simulink model "satellite_dynamics"  (R2025a)
settings: Solver=ode4  StartTime=0.0  StopTime=5400* 5  FixedStep=gyro.Ts  RelTol=1e-6
values from neighbouring files (symbols this model uses):
  altitude = 279e3    (= 279000)    [orbit_params.m]
  G = 6.674e-11    [orbit_params.m]    (also in update_MEKF_new.m = [-eye(3,3), zeros(3,3),zeros(3,3);          zeros(3,3), eye(; update_MEKF_old.m = [-eye(3,3), zeros(3,3);          zeros(3,3), eye(3,3)]; wheel_analysis.m = [ D)
  h_default = h_default + wheel.omega_initial(f) *  wheel.I_II * wheel.axes(:,f)    [orbit_params.m]
  K = convhulln(V)    [wheel_analysis.m]
  m = size(A, 2)    [wheel_analysis.m]
  omega_icrf2b_initial = [-0.3804;-0.2976;0.06] *0    [orbit_params.m]
  P_initial = blkdiag(eye(3) * gyro.sigma_v^2 * 1e4 ,eye(3) * gyro.sigma_u^2 * 1e5)    [orbit_params.m]
  Q_c = blkdiag(eye(3) * gyro.sigma_v^2/2 ,eye(3) * gyro.sigma_u^2/2 )    [orbit_params.m]
  q_icrf2b_initial = q_icrf2b_initial/norm(q_icrf2b_initial)    [orbit_params.m]
  q_initial = q_icrf2b_initial    [orbit_params.m]
  R_k_star = blkdiag(star.sigma_cross^2,star.sigma_cross^2,star.sigma_bore^2) * ((1/3600) * pi/180)^2    [orbit_params.m]
  r_offset = [1;1;5] * 1e-2    [orbit_params.m]
  regulation_kp = regulation.kp    [orbit_params.m]
  s = sign(h_bias)    [min_h.m]
  Ts = 0.1    [orbit_params.m]    (also in untitled2.m = 0.005)
  x_initial = zeros(6,1)    [orbit_params.m]
undefined symbols (not defined in the file or in its folder): DiscIntNeverNeededParam, earth, gyro, Kalman, mag, mag_torque, NEO, regulation, star, sun, tracking, wheel
libraries: utilities x24, simulink_extras x21, aerolibutil x20, dspmathops x19, matrix_library x9, simulink x8, dspstat3 x8, sharedutil x3, aerolibgravity2 x1, eeGeneralControl x1
(part 1 of 2)
settings Model: PacingRate=0.100000  Creator=OlguPilav  LastModifiedBy=OlguPilav

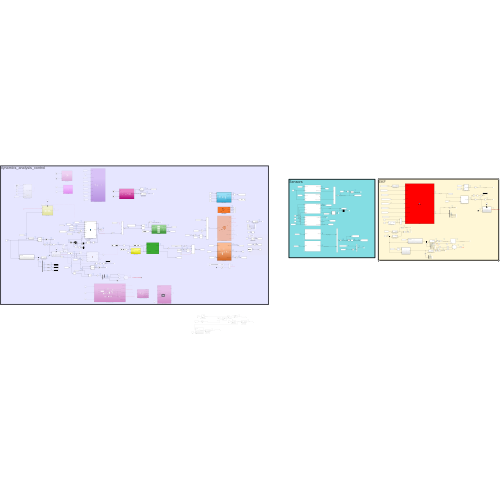
[thumbnail: Simulink's stored preview of the top-level diagram]
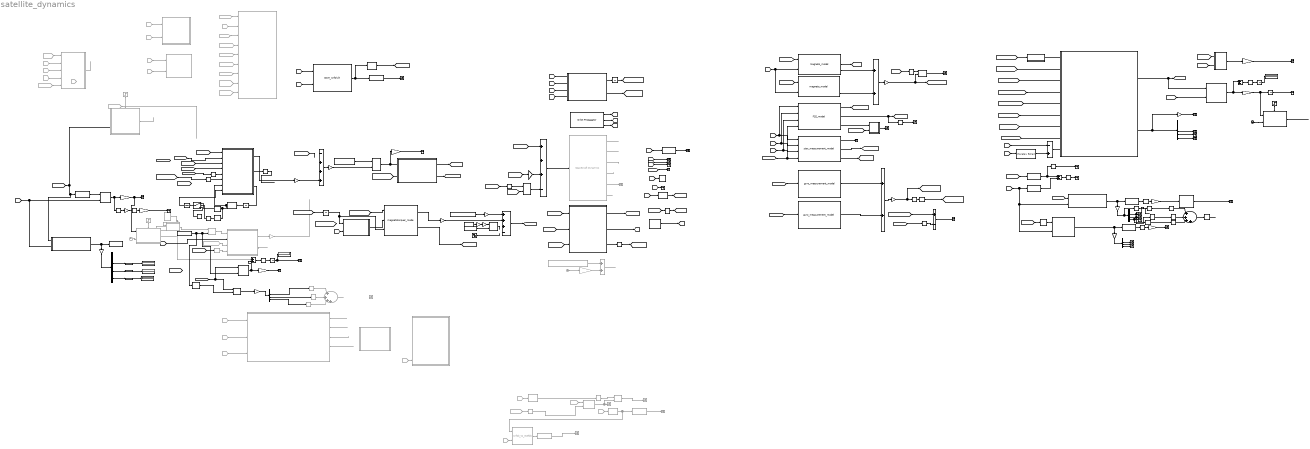
== system satellite_dynamics ==
  note: EKF
  note: Sensors
  note: dynamics_analysis_control
  Abs{,1..5} (6 alike) : Abs  SaturateOnIntegerOverflow=off
  Add : Sum
  Bias : Bias  Bias=gyro.bias  SaturateOnIntegerOverflow=off
  Clock : Clock  Commented=on
  Clock1 : Clock  Commented=on
  Clock2 : Clock
  Compare To Constant : simulink/Logic and Bit Operations/Compare To Constant  relop=>  const=0.999999  OutDataTypeStr=boolean
  Constant : Constant  Commented=on  Value=juliandate(year, month, day, hour, minute, second)
  Constant1 : Constant  Value=r_offset
  Constant2 : Constant  Value=q_icrf2b_initial
  Constant3 : Constant  Value=[0;0;0]
  Constant4 : Constant  Commented=on  Value=[1;1;1]
  Constant5 : Constant  Commented=on  Value=0
  Constant7 : Constant  Value=wheel.distribution_matrix
  Cross Product : matrix_library/Cross Product
  Cross Product1 : matrix_library/Cross Product
  DCM_icrf2lvlh : utilities/DCM_icrf2lvlh  SystemSampleTime=-1  VariantActivationTime=update diagram  EmptyChoice=off  PassThrough=off  PassThroughVariantControl=(default)  EmptyChoiceVariantControl=(default)  AllowFlexibleInterface=on  Latency=0  AutoFrameSizeCalculation=off
  Degrees to Radians : simulink_extras/Transformations/Degrees to Radians  Commented=on
  Degrees to Radians{1..6} (6 alike) : simulink_extras/Transformations/Degrees to Radians
  Degrees to Radians7 : simulink_extras/Transformations/Degrees to Radians  Commented=on
  Demux : Demux  Outputs=6
  Demux{1..4} (4 alike) : Demux
  Derivative : Derivative
  Direction Cosine Matrix to Rotation Angles : Dcm2Angle  Commented=on
      settings: AttributesFormatString=Rotation Order: %<rotationOrder>
  Direction Cosine Matrix to Rotation Angles1 : Dcm2Angle  Commented=on
      settings: AttributesFormatString=Rotation Order: %<rotationOrder>
  Direction Cosine Matrix to Rotation Angles2 : Dcm2Angle
      settings: AttributesFormatString=Rotation Order: %<rotationOrder>
  Direction Cosine Matrix to Quaternions : Dcm2Quat
  Direction Cosine Matrix to Quaternions1 : Dcm2Quat
  Discrete-Time Integrator : DiscreteIntegrator  SampleTime=-1  ICPrevOutput=DiscIntNeverNeededParam  ICPrevScaledInput=DiscIntNeverNeededParam
  Display{,1..4} (5 alike) : Display
  FSS_model : utilities/FSS_model  sun=sun
  Feedforward_torque_legacy : Subsystem  Commented=on
  From Workspace : FromWorkspace  VariableName=drag_simin
  From10 : From  Commented=on  GotoTag=omegaicrf2b_b
  From12 : From  Commented=on  GotoTag=tutc
  From13 : From  Commented=on  GotoTag=tutc
  From{14,20,43,83,96} (5 alike) : From  Commented=on  GotoTag=inertia
  From15 : From  Commented=on  GotoTag=Xicrf
  From{6,9,16,19,27..28,64} (7 alike) : From  Commented=on  GotoTag=qicrf2b
  From18 : From  Commented=on  GotoTag=omegaicrf2b_b
  From44 : From  Commented=on  GotoTag=Xicrf
  From45 : From  Commented=on  GotoTag=Vicrf
  From47 : From  Commented=on  GotoTag=DCMicrf2b
  From52 : From  Commented=on  GotoTag=DCMicrf2b
  From53 : From  Commented=on  GotoTag=hwheelsbody
  From{60..63} (4 alike) : From  Commented=on  GotoTag=dcmb2icrf
  From66 : From  Commented=on  GotoTag=Xicrf
  From84 : From  Commented=on  GotoTag=hwheelsbody
  From85 : From  Commented=on  GotoTag=q_icrf2b_kalman
  From93 : From  Commented=on  GotoTag=hwheelsbody
  Gain : Gain  Gain=0
  Gain1 : Gain  Gain=1/2
  Gain10 : Gain  Gain=3600 * 2 * 180/pi
  Gain11 : Gain  Gain=3600 * 2 * 180/pi
  Gain12 : Gain  Gain=1000
  Gain13 : Gain  Commented=on  Gain=1/86400
  Gain14 : Gain  Gain=3600 * 180/pi
  Gain15 : Gain  Gain=altitude
  Gain16 : Gain  Gain=1/2
  Gain17 : Gain  Gain=[-1;0;0]
  Gain18 : Gain  Gain=3600 * 2 * 180/pi
  Gain{2..3,6,8..9,19} (6 alike) : Gain  Gain=3600
  Gain20 : Gain  Gain=(2 * 180/pi) * 3600
  Gain21 : Gain  Commented=on
  Gain22 : Gain
  Gain23 : Gain  Gain=0
  Gain24 : Gain
  Gain4 : Gain  Gain=-1
  Gain5 : Gain  Gain=1/2
  Gain7 : Gain
  Integrator : Integrator
  Integrator1 : Integrator
  Integrator2 : Integrator
  MATLAB Function : MATLAB Function  Commented=on  TreatAsAtomicUnit=on
  MATLAB Function1 : MATLAB Function  TreatAsAtomicUnit=on
  MEKF : MATLAB Function  TreatAsAtomicUnit=on  SystemSampleTime=Kalman.Ts
  Matrix Multiply4 : Product  Multiplication=Matrix(*)
  Matrix Multiply7 : Product  Multiplication=Matrix(*)
  Matrix Multiply8 : Product  Commented=on  Multiplication=Matrix(*)
  Matrix Multiply9 : Product  Commented=on  Multiplication=Matrix(*)
  Moving Variance : dspstat3/Moving Variance  Method=Sliding window  ForgettingFactorPort=off  SpecifyWindowLength=on  WindowLength=20000  OverlapLength=19999  AllowArbitraryInputLength=off  ForgettingFactor=0.9  SimulateUsing=Interpreted execution
  Moving Variance1 : dspstat3/Moving Variance  Method=Sliding window  ForgettingFactorPort=off  SpecifyWindowLength=on  WindowLength=20000  OverlapLength=19999  AllowArbitraryInputLength=off  ForgettingFactor=0.9  SimulateUsing=Interpreted execution
  Moving Variance2 : dspstat3/Moving Variance  Method=Sliding window  ForgettingFactorPort=off  SpecifyWindowLength=on  WindowLength=20000  OverlapLength=19999  AllowArbitraryInputLength=off  ForgettingFactor=0.9  SimulateUsing=Interpreted execution
  Moving Averaage : Subsystem
  Orbit Propagator Kepler (unperturbed) : OrbitPropagator  startDate=juliandate(year, month, day, hour, minute, second)  semiMajorAxis=semi_major  eccentricity=eccentricity  inclination=inclination  raan=RAAN  argPeriapsis=periapsis_arg  trueAnomaly=true_anomaly  inertialPosition=[3649700.0 3308200.0 -4676600.0]  inertialVelocity=[-2750.8 6666.4 2573.4]  fixedPosition=[-4142689.0 -2676864.7 -4669861.6]  fixedVelocity=[1452.7 -6720.7 2568.1]  customR=3396200  customMu=4.305e13  customJ2=1.0826269e-03  customOmega=4.06125949e-3
  Planetary Ephemeris : PlanetaryEphem  units=m,m/s  target=Sun  outputVelocity=off
  Quaternion Inverse : aerolibutil/Quaternion Inverse
  Quaternion Inverse2 : aerolibutil/Quaternion Inverse
  Quaternion Multiplication : aerolibutil/Quaternion Multiplication  Commented=on
  Quaternion Multiplication1 : aerolibutil/Quaternion Multiplication
  Quaternions to Direction Cosine Matrix : Quat2Dcm  Commented=on
  Quaternions to Direction Cosine Matrix1 : Quat2Dcm
  Quaternions to Direction Cosine Matrix2 : Quat2Dcm  Commented=on
  Quaternions to Rotation Angles{,1..5} (6 alike) : Quat2Angle
      settings: AttributesFormatString=Rotation Order: %<rotationOrder>
  Radians to Degrees{,1..4} (5 alike) : simulink_extras/Transformations/Radians to Degrees
  Selector : Selector  InputPortWidth=4  IndexOptions=Index vector (dialog)  Indices=[2:4]  OutputSizes=1
  Selector1 : Selector  InputPortWidth=4  IndexOptions=Index vector (dialog)  Indices=[1]  OutputSizes=1
  Sine Wave : Sin  Amplitude=0.001  Frequency=6  SampleTime=0
  Spacecraft Dynamics : SpacecraftDynamics  Commented=on  forcesIn=off  startDate=juliandate(year, month, day, hour, minute, second)  mass=NEO.mass  inertia=NEO.inertia  semiMajorAxis=semi_major  eccentricity=eccentricity  inclination=inclination  raan=RAAN  argPeriapsis=periapsis_arg  trueAnomaly=true_anomaly  attitude=q_icrf2b_initial  attitudeRate=omega_icrf2b_initial  outputAngAccel=on  useGravGrad=off  useEOPs=off  useThirdBodyGravity=on  useSRP=on
  Sqrt : Sqrt
  Square : Math  Operator=square
  Square1 : Math  Operator=square
  Square2 : Math  Operator=square
  Square3 : Math  Commented=on  Operator=square
  Square4 : Math  Commented=on  Operator=square
  Square5 : Math  Commented=on  Operator=square
  Step : Step  Commented=on  SampleTime=0
  Step1 : Step  Commented=on  Time=1000  SampleTime=0
  Step2 : Step  Time=1000  SampleTime=0
  Subsystem : Subsystem  Commented=on
  Subsystem1 : Subsystem
  Subsystem2 : Subsystem  TreatAsAtomicUnit=on  SystemSampleTime=star.Ts
  Subsystem3 : Subsystem  TreatAsAtomicUnit=on  SystemSampleTime=Kalman.Ts
  Subsystem4 : Subsystem
  Subsystem6 : Subsystem  TreatAsAtomicUnit=on  SystemSampleTime=Kalman.Ts
  Subtract{,1,3..4} (4 alike) : Sum  Inputs=+-
  Subtract2 : Sum  Inputs=-+
  Sum : Sum
  Sum of Elements : Sum  Inputs=+
  Sum1 : Sum  Inputs=-+++
  Sum2 : Sum  Commented=on
  Sum3 : Sum  Inputs=|++++
  Sum4 : Sum  Commented=on  Inputs=|++++
  Sum6 : Sum  Inputs=+++-
  Sum7 : Sum  Inputs=+++-
  Switch : Switch  Criteria=u2 > Threshold  SaturateOnIntegerOverflow=off  InputSameDT=off
  Tan : Trigonometry  Operator=tan
  Terminator{,1..3,5..6,9..13,16..36,38} (33 alike) : Terminator
  Terminator{4,7..8,14..15,37} (6 alike) : Terminator  Commented=on
  Transpose2 : Math  Operator=transpose
  Transpose4 : Math  Operator=transpose
  Transpose5 : Math  Commented=on  Operator=transpose
  Unit Delay : UnitDelay  SampleTime=-1  HasFrameUpgradeWarning=on
  Unit Delay1 : UnitDelay  InitialCondition=[50,50,50]  SampleTime=-1  HasFrameUpgradeWarning=on
  Unit Delay2 : UnitDelay  InitialCondition=[50,50,50]  SampleTime=-1  HasFrameUpgradeWarning=on
  angular_momentum_calculations : Subsystem  Commented=on
  average_angle_knowledge_error : Subsystem  AncestorBlock=utilities/average_angle_knowledge_error  TreatAsAtomicUnit=on  SystemSampleTime=Kalman.Ts  mask{samples=2}
  average_angle_knowledge_error1 : Subsystem  AncestorBlock=utilities/average_angle_knowledge_error  TreatAsAtomicUnit=on  SystemSampleTime=star.Ts  mask{samples=2}
  average_angle_knowledge_error2 : utilities/average_angle_knowledge_error  samples=2
  average_angle_knowledge_error3 : utilities/average_angle_knowledge_error  samples=2
  disturbance : Constant  Value=[0.00001,0.00005,0.000]'  VectorParams1D=off
  earth_tracking_controller : MATLAB Function  TreatAsAtomicUnit=on
  geo_constrained_prograde aligned : Subsystem  Commented=on
  gyro_measurement_model : utilities/gyro_measurement_model  omega_initial=omega_icrf2b_initial  gyro=gyro
  gyro_measurement_model1 : utilities/gyro_measurement_model  omega_initial=omega_icrf2b_initial  gyro=gyro2
  icrf2b_to_ecef2b : utilities/icrf2b_to_ecef2b  Commented=on  SystemSampleTime=-1  VariantActivationTime=update diagram  EmptyChoice=off  PassThrough=off  PassThroughVariantControl=(default)  EmptyChoiceVariantControl=(default)  AllowFlexibleInterface=on  Latency=0  AutoFrameSizeCalculation=off
  inertia_b : Constant  Value=NEO.inertia
  magnetic_field_slow : Subsystem  TreatAsAtomicUnit=on  SystemSampleTime=60
  magneto_model : utilities/magneto_model  mag=mag
  magneto_model1 : utilities/magneto_model  mag=mag2
  magnetotorquer_mode : utilities/magnetotorquer_mode  Parameter1=mag_torque
  magtor_controller : Subsystem
  nadir_constrained_sun_aligned : Subsystem  Commented=on
  olgus_dynamics : Subsystem  TreatAsAtomicUnit=on  SystemSampleTime=Ts
  quat_tester : Subsystem  Commented=on
  quat_tester_2 : Subsystem  Commented=on
  regulating_controller : MATLAB Function  Commented=on  TreatAsAtomicUnit=on  SystemSampleTime=Kalman.Ts
  star_measurement_model : utilities/star_measurement_model  star=star
  target_q_generator : Subsystem  Commented=on
  vector_magnitude : utilities/vector_magnitude
  vector_magnitude1 : utilities/vector_magnitude
  wheel_controller : Subsystem  Commented=on  TreatAsAtomicUnit=on  SystemSampleTime=Kalman.Ts
  wheels_dynamics : Subsystem
  wires:
  Spacecraft Dynamics/5 -> Terminator4/1  "omega_dot_icrf2b"
  Quaternions to Direction Cosine Matrix/1 -> Direction Cosine Matrix to Rotation Angles/1, icrf2b_to_ecef2b/1  "DCM_icrf2b"
  icrf2b_to_ecef2b/1 -> Direction Cosine Matrix to Rotation Angles1/1
  Direction Cosine Matrix to Rotation Angles/1 -> Terminator7/1  "R_icrf2b"
  Direction Cosine Matrix to Rotation Angles1/1 -> Terminator8/1  "R_ecef2b"
  Spacecraft Dynamics/1 -> ?  "X_icrf"
  [Xicrf] -> Terminator/1
  Spacecraft Dynamics/2 -> ?  "V_icrf"
  [Vicrf] -> Terminator1/1
  Spacecraft Dynamics/3 -> ?  "q_icrf2b"
  [qicrf2b] -> Terminator2/1
  From6/1 -> Quaternions to Direction Cosine Matrix/1
  Spacecraft Dynamics/4 -> ?  "omega_icrf2b_b"
  [omegaicrf2b_b] -> Terminator3/1
  Spacecraft Dynamics/6 -> ?  "t_utc"
  [tutc] -> Terminator5/1
  From13/1 -> icrf2b_to_ecef2b/2
  inertia_b/1 -> [inertia]  "inertia"
  [qicrf2b] -> Quaternions to Direction Cosine Matrix1/1
  From19/1 -> Quaternions to Direction Cosine Matrix2/1
  Quaternions to Direction Cosine Matrix2/1 -> Transpose5/1  "DCM_icrf2b"
  From18/1 -> Degrees to Radians/1
  Matrix Multiply9/1 -> Matrix Multiply8/2, Terminator14/1  "h_body"
  Transpose5/1 -> Matrix Multiply8/1
  Matrix Multiply8/1 -> Terminator15/1  "h_icrf2"
  Degrees to Radians/1 -> Matrix Multiply9/2  "omega_body"
  From20/1 -> Matrix Multiply9/1
  [Xicrf] -> DCM_icrf2lvlh/1
  [Vicrf] -> DCM_icrf2lvlh/2
  DCM_icrf2lvlh/1 -> Direction Cosine Matrix to Quaternions/1, Direction Cosine Matrix to Rotation Angles2/1  "DCM_icrf2lvlh"
  Direction Cosine Matrix to Rotation Angles2/1 -> Terminator6/1  "R_LVLH"
  [qicrf2b] -> Quaternions to Rotation Angles/1
  Quaternions to Rotation Angles/1 -> Terminator9/1  "R_icrf"
  Direction Cosine Matrix to Quaternions/1 -> [qicrf2lvlh]  "q_icrf2lvlh"
  From16/1 -> nadir_constrained_sun_aligned/2(In2)
  From15/1 -> nadir_constrained_sun_aligned/1(In1)
  From12/1 -> nadir_constrained_sun_aligned/3(In3)
  nadir_constrained_sun_aligned/1(tar_primary_icrf) -> ?
  nadir_constrained_sun_aligned/2(tar_secondary_icrf) -> ?
  nadir_constrained_sun_aligned/3(body_primary_icrf) -> ?
  nadir_constrained_sun_aligned/4(body_secondary_icrf) -> ?
  From9/1 -> target_q_generator/5(qicrf2b)
  [qicrf2b] -> vector_magnitude1/1
  olgus_dynamics/1(omega_icrf2b_b) -> [omegaicrf2b_b]  "omega_icrf2b_b_new"
  olgus_dynamics/2(q_icrf2b) -> [qicrf2b]  "q_icrf2b"
  [omegaicrf2b_b] -> gyro_measurement_model/1
  gyro_measurement_model/1 -> Sum/1  "omega_icrf2b_gyro"
  [Xicrf] -> star_measurement_model/2, FSS_model/2
  [tutc] -> FSS_model/3, star_measurement_model/3
  star_measurement_model/1 -> Terminator13/1  "q_icrf2star_meas"
  [qicrf2b] -> FSS_model/1, star_measurement_model/1
  [omegaicrf2b_b] -> gyro_measurement_model1/1
  gyro_measurement_model1/1 -> Sum/2  "omega_icrf2b_gyro2"
  Sum/1 -> Gain1/1
  Gain1/1 -> [omega_gyro_pre_bias_degree], Degrees to Radians3/1  "omega_icrf2b_gyro_mean"
  MEKF/1(q_k_k) -> average_angle_knowledge_error/1(q_1), [q_icrf2b_kalman]  "q_icrf2b_kalman"
  MEKF/2(x_k_k) -> Gain14/1, Demux/1  "x_kalman"
  [omegaicrf2b_b] -> Degrees to Radians4/1
  Degrees to Radians4/1 -> Subtract1/2
  Subtract1/1 -> ?  "bias"
  Demux/4 -> Terminator26/1  "bias_kalman_1"
  Demux/5 -> Terminator28/1  "bias_kalman_2"
  Demux/6 -> Terminator27/1  "bias_kalman_3"
  [qicrf2b] -> average_angle_knowledge_error/2(q_2)
  average_angle_knowledge_error/1(error_degrees) -> Subtract4/1, Gain3/1  "error_kalman"
  [qicrf2b] -> average_angle_knowledge_error1/2(q_2)
  average_angle_knowledge_error1/1(error_degrees) -> Gain2/1  "error_star"
  Gain3/1 -> Subsystem4/1(In1), Integrator1/1  "error_kalman_arcsec"
  Gain2/1 -> Terminator18/1  "error_star_arcsec"
  Integrator1/1 -> Terminator16/1  "integral_kalman_error"
  [Xicrf] -> Subtract2/1
  [tutc] -> Planetary Ephemeris/1
  Planetary Ephemeris/1 -> Subtract2/2  "sun_icrf"
  Subtract2/1 -> MEKF/9(sat2sun_icrf)  "sat2sun_icrf"
  Sum of Elements/1 -> Terminator24/1
  [qicrf2b] -> magneto_model1/2, magneto_model/2
  magneto_model/3 -> Add/1
  magneto_model1/3 -> Add/2
  Add/1 -> Gain5/1
  Gain5/1 -> Matrix Multiply4/2, [magXYZbodymeasavg]  "mag_XYZ_body_meas_avg"
  [DCMicrf2b] -> Transpose2/1
  Transpose2/1 -> Matrix Multiply4/1
  Matrix Multiply4/1 -> Terminator11/1  "mag_XYZ_icrf_meas_avg"
  Gain6/1 -> Subsystem/1(In1), Terminator21/1  "error_target_arcsec"
  average_angle_knowledge_error2/1 -> Degrees to Radians1/1, Gain6/1  "error_target"
  earth_tracking_controller/1(torque) -> Gain24/1
  Sum1/1 -> Gain7/1
  Quaternions to Rotation Angles1/1 -> Subtract3/1, Radians to Degrees1/1
  Quaternions to Rotation Angles2/1 -> Subtract3/2
  Subtract3/1 -> Radians to Degrees/1
  Radians to Degrees/1 -> Terminator17/1
  Radians to Degrees1/1 -> Terminator19/1  "rot_angles_est"
  Gain7/1 -> Matrix Multiply7/2
  Degrees to Radians3/1 -> Bias/1
  Quaternions to Rotation Angles3/1 -> Radians to Degrees2/1  "rot_errors"
  Gain8/1 -> vector_magnitude/1  "rot_errors_kalman_arcsec"
  Radians to Degrees2/1 -> Gain8/1
  Quaternions to Rotation Angles4/1 -> Radians to Degrees3/1
  Gain9/1 -> Terminator31/1  "rot_errors_star_arcsec"
  [qicrf2b] -> Quaternions to Rotation Angles2/1, Subsystem2/2(r), Subsystem3/2(r)
  Radians to Degrees3/1 -> Gain9/1
  Demux2/4 -> Terminator35/1  "z_star"
  Demux3/2 -> Abs1/1, Terminator29/1  "x_k"
  Demux3/3 -> Abs2/1, Terminator30/1  "y_k"
  Demux3/4 -> Abs3/1, Terminator32/1  "z_k"
  Demux2/3 -> Terminator34/1  "y_star"
  Demux2/2 -> Terminator33/1  "x_star"
  Gain10/1 -> Abs/1, Demux3/1
  Gain11/1 -> Demux2/1
  Subsystem2/1(q*r) -> Gain11/1, Quaternions to Rotation Angles4/1
  Quaternion Inverse2/1 -> Subsystem2/1(q)
  Subsystem3/1(q*r) -> Quaternions to Rotation Angles3/1, Gain10/1
  Moving Averaage/1(omega_movav) -> MEKF/1(omega_icrf2b_gyro)
  FSS_model/2 -> [FSSvalid], Sum of Elements/1  "FSS_valid"
  Gain14/1 -> Terminator12/1  "x_kalman_arcsec"
  vector_magnitude/1 -> Terminator25/1  "mag_error_kalman_rot"
  FSS_model/3 -> MATLAB Function1/1(b1)
  MATLAB Function1/1(y) -> Terminator23/1  "vars"
  Constant7/1 -> Matrix Multiply7/1
  Matrix Multiply7/1 -> Gain12/1, wheels_dynamics/1(wheel_torques)
  [omega_dot_body] -> wheels_dynamics/2(satellite_body_omega_dot)
  Gain4/1 -> Sum6/3
  Gain12/1 -> Terminator20/1  "wheel_torques_demand_mNm"
  olgus_dynamics/3(omega_dot_icrf2b_b) -> Degrees to Radians5/1
  Degrees to Radians5/1 -> [omega_dot_body]
  Step/1 -> wheel_controller/Enable
  ? -> wheel_controller/1(qicrf2b)
  Subsystem1/1(q_out) -> average_angle_knowledge_error2/1
  Sum6/1 -> Spacecraft Dynamics/1
  Cross Product1/1 -> Sum6/4
  Degrees to Radians2/1 -> Cross Product1/1
  [mag_XYZ_b_model] -> magnetotorquer_mode/1
  magnetotorquer_mode/1 -> Gain23/1
  magtor_controller/1(currents) -> magnetotorquer_mode/2
  [magXYZbodymeasavg] -> Unit Delay2/1
  disturbance/1 -> Gain/1
  Gain/1 -> Sum7/1
  wheels_dynamics/2(angular_momentum_body) -> [hwheelsbody]  "h_wheels_body"
  [hwheelsbody] -> Cross Product1/2
  [hwheelsbody] -> olgus_dynamics/2(h_wheels_body)
  [hwheelsbody] -> magtor_controller/2(h_wheels_body)
  From44/1 -> Feedforward_torque_legacy/2(Xicrf)
  From45/1 -> Feedforward_torque_legacy/3(Vicrf)
  Feedforward_torque_legacy/1(target_torque) -> ?
  Quaternions to Direction Cosine Matrix1/1 -> [DCMicrf2b]  "DCM_icrf2b"
  [DCMicrf2b] -> Transpose4/1
  From52/1 -> Feedforward_torque_legacy/1(DCM_icrf2b)
  wheels_dynamics/1(body_torque) -> [wheelsbodytorque]  "wheels_body_torque"
  [wheelsbodytorque] -> olgus_dynamics/1(Mb_wheel)
  [wheelsbodytorque] -> Gain4/1
  Sum7/1 -> [Mbexternal]  "Mb_external"
  [Mbexternal] -> olgus_dynamics/3(Mb_external)
  [Mbexternal] -> Sum6/1
  [omegaicrf2b_b] -> Degrees to Radians2/1
  Transpose4/1 -> [dcmb2icrf]  "dcm_b2icrf"
  From28/1 -> quat_tester/1(q)
  From64/1 -> quat_tester/2(In2)
  From62/1 -> angular_momentum_calculations/1(dcmb2icrf)
  From43/1 -> angular_momentum_calculations/2(inertia)
  From10/1 -> angular_momentum_calculations/3(omegaicrf2b_b)
  From60/1 -> angular_momentum_calculations/4(dcmb2icrf2)
  From14/1 -> angular_momentum_calculations/5(inertia2)
  From47/1 -> angular_momentum_calculations/6(DCMicrf2b)
  From63/1 -> angular_momentum_calculations/7(dcmb2icrf3)
  From61/1 -> angular_momentum_calculations/8(dcmb2icrf4)
  From53/1 -> angular_momentum_calculations/9(hwheelsbody)
  From27/1 -> quat_tester_2/1(In1)
  From66/1 -> quat_tester_2/2(X_icrf)
  [magXYZicrfmodel] -> MATLAB Function1/2(b2)
  [magXYZicrfmodel] -> MEKF/6(mag_XYZ_icrf_model)
  [magXYZicrfmodel] -> magneto_model1/1
  [magXYZicrfmodel] -> magneto_model/1
  Bias/1 -> [omegaicrf2bgyromeanrad]  "omega_icrf2b_gyro_mean_rad"
  [omegaicrf2bgyromeanrad] -> Moving Averaage/1(omega_in)
  [omegaicrf2bgyromeanrad] -> Subtract1/1
  magneto_model/2 -> [magvalid]  "mag_valid"
  [magvalid] -> MEKF/8(mag_valid)
  [magXYZbodymeasavg] -> MEKF/7(mag_XYZ_body_meas)
  FSS_model/1 -> [sat2sunbody]  "sat2sun_body"
  [sat2sunbody] -> MEKF/4(sun_vectors)
  [FSSvalid] -> MEKF/5(sun_valid)
  star_measurement_model/3 -> [qicrf2bstartracker]  "q_icrf2b_star_tracker"
  [qicrf2bstartracker] -> MEKF/2(q_icrf2b_star)
  [qicrf2bstartracker] -> average_angle_knowledge_error1/1(q_1)
  [qicrf2bstartracker] -> Quaternion Inverse2/1
  [q_icrf2b_kalman] -> Quaternions to Rotation Angles1/1
  [q_icrf2b_kalman] -> Subsystem3/1(q_icrf2b_kalman)
  From83/1 -> Feedforward_torque_legacy/4(inertia)
  From84/1 -> Feedforward_torque_legacy/5(hwheelsbody)
  [qicrf2b] -> magnetic_field_slow/1(In1)
  [Xicrf] -> magnetic_field_slow/2(vector_icrf)
  [tutc] -> magnetic_field_slow/3(t_utc)
  [tutc] -> magnetic_field_slow/4(t_utc1)
  magnetic_field_slow/1(mag_XYZ_b_model) -> Unit Delay1/1
  magnetic_field_slow/2(mag_XYZ_icrf_model) -> [magXYZicrfmodel]
  Clock/1 -> Gain13/1
  Sum2/1 -> ?
  Gain13/1 -> Sum2/2
  Constant/1 -> Sum2/1
  Orbit Propagator Kepler (unperturbed)/1 -> [Xicrf]  "X_icrf"
  Orbit Propagator Kepler (unperturbed)/2 -> [Vicrf]  "V_icrf"
  Orbit Propagator Kepler (unperturbed)/3 -> [tutc]
  Degrees to Radians1/1 -> Gain16/1
  Tan/1 -> Gain15/1
  Gain15/1 -> Terminator36/1  "error_geo_meter"
  Gain16/1 -> Tan/1
  star_measurement_model/2 -> [STARVALID]  "STAR_VALID"
  [STARVALID] -> MEKF/3(star_valid)
  Cross Product/1 -> ?
  From Workspace/1 -> Gain22/1
  Constant1/1 -> Cross Product/2
  Gain17/1 -> Cross Product/1
  [qicrf2lvlh] -> earth_tracking_controller/1(q_icrf2lvlh)
  From85/1 -> ?
  [Xicrf] -> earth_tracking_controller/3(X_icrf)
  [Vicrf] -> earth_tracking_controller/4(V_icrf)
  [Vicrf] -> Derivative/1
  Derivative/1 -> earth_tracking_controller/5(V_icrf_dot)
  [omega_gyro_pre_bias_degree] -> Degrees to Radians6/1
  earth_tracking_controller/2(omega_c) -> Radians to Degrees4/1
  wheel_controller/1(wheel_torque) -> ?
  Degrees to Radians6/1 -> earth_tracking_controller/6(omega_b)
  Radians to Degrees4/1 -> ?
  earth_tracking_controller/3(dA) -> Unit Delay/1
  Direction Cosine Matrix to Quaternions1/1 -> Selector1/1, Selector/1, earth_tracking_controller/7(dq)
  Unit Delay/1 -> Direction Cosine Matrix to Quaternions1/1
  Unit Delay1/1 -> [mag_XYZ_b_model]
  Step1/1 -> Subsystem/Enable
  Subsystem/1(Out1) -> ?  "error_target_arcsec_mean"
  Clock1/1 -> Subsystem/2(In2)
  Step2/1 -> Subsystem4/Enable
  Clock2/1 -> Subsystem4/2(In2)
  Subsystem4/1(Out1) -> ?  "error_kalman_arcsec_mean"
  Abs/1 -> ?
  Sum3/1 -> Sqrt/1
  Abs1/1 -> Square/1
  Abs2/1 -> Square1/1
  Abs3/1 -> Square2/1
  Square/1 -> Sum3/1
  Square2/1 -> Sum3/3
  Square1/1 -> Sum3/2
  Sqrt/1 -> ?
  [qicrf2b] -> Subsystem6/2(r), average_angle_knowledge_error2/2
  [qicrf2lvlh] -> wheel_controller/2(qicrf2lvlh), Subsystem6/1(q_icrf2b_kalman), Subsystem1/1(q)
  Subsystem6/1(q*r) -> Quaternions to Rotation Angles5/1, Gain18/1
  Demux1/4 -> Moving Variance2/1  "z_tar"
  Gain18/1 -> Demux1/1
  Demux1/3 -> Moving Variance1/1  "y_tar"
  Demux1/2 -> Moving Variance/1  "x_tar"
  Sine Wave/1 -> ?
  From93/1 -> regulating_controller/3(hwheelsbody)
  Degrees to Radians7/1 -> regulating_controller/4(omega_b)
  regulating_controller/2(dq) -> ?  "regulation_dq"
  Quaternion Multiplication/1 -> regulating_controller/1(q_icrf2tar)
  MATLAB Function/1(quat) -> Quaternion Multiplication/1
  Constant4/1 -> MATLAB Function/2(vector)
  average_angle_knowledge_error3/1 -> Subtract/2, Gain19/1  "error_target"
  Gain19/1 -> Terminator22/1  "error_target_arcsec"
  [q_icrf2b_kalman] -> earth_tracking_controller/2(q_icrf2b)
  Constant5/1 -> Subtract/1, MATLAB Function/1(angle_deg)
  Constant2/1 -> Quaternion Inverse/1, average_angle_knowledge_error3/2, Quaternion Multiplication/2
  [qicrf2b] -> average_angle_knowledge_error3/1, Quaternion Multiplication1/1
  Quaternion Inverse/1 -> Quaternion Multiplication1/2
  Square5/1 -> Sum4/3
  Square3/1 -> Sum4/1
  Demux4/4 -> Square5/1  "z"
  Quaternion Multiplication1/1 -> Gain20/1
  Demux4/3 -> Square4/1  "y"
  Square4/1 -> Sum4/2
  Demux4/2 -> Square3/1  "x"
  ? -> Terminator37/1
  Sum4/1 -> ?
  Gain20/1 -> Demux4/1
  Subtract/1 -> Abs4/1
  Abs4/1 -> Integrator/1
  Integrator/1 -> Display/1, Terminator38/1  "integral_error"
  regulating_controller/1(torque) -> Gain21/1
  [omegaicrf2b_b] -> Degrees to Radians7/1
  Abs5/1 -> Integrator2/1
  Integrator2/1 -> Display1/1  "integral_error"
  Subtract4/1 -> Abs5/1
  Gain21/1 -> ?
  Gain22/1 -> Gain17/1
  [qicrf2b] -> regulating_controller/2(q_icrf2b)
  Gain23/1 -> Sum7/2
  [mag_torque] -> ?
  Selector/1 -> Switch/1
  Discrete-Time Integrator/1 -> earth_tracking_controller/8(dq_int)
  Switch/1 -> Discrete-Time Integrator/1
  Selector1/1 -> Compare To Constant/1
  Compare To Constant/1 -> Switch/2
  Constant3/1 -> Switch/3
  [omegaicrf2b_b] -> star_measurement_model/4, FSS_model/4
  magnetotorquer_mode/2 -> [mag_torque]
  Unit Delay2/1 -> magnetotorquer_mode/3, magtor_controller/1(mag_XYZ_body)
  Moving Variance/1 -> Display2/1
  Moving Variance2/1 -> Display4/1
  Moving Variance1/1 -> Display3/1
  Gain24/1 -> Sum1/4

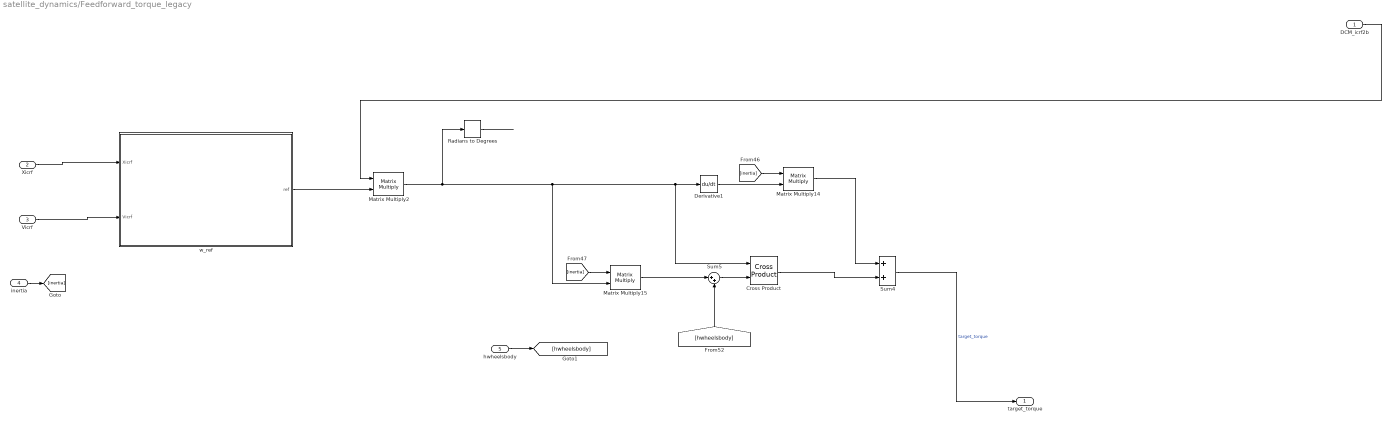
== system satellite_dynamics/Feedforward_torque_legacy ==
  DCM_icrf2b : Inport
  Xicrf : Inport  Port=2
  Vicrf : Inport  Port=3
  inertia : Inport  Port=4
  hwheelsbody : Inport  Port=5
  Cross Product : matrix_library/Cross Product
  Derivative1 : Derivative
  Matrix Multiply14 : Product  Multiplication=Matrix(*)
  Matrix Multiply15 : Product  Multiplication=Matrix(*)
  Matrix Multiply2 : Product  Multiplication=Matrix(*)
  Radians to Degrees : simulink_extras/Transformations/Radians to Degrees
  Sum4 : Sum
  Sum5 : Sum  Inputs=|++
  w_ref : Subsystem
  target_torque : Outport
  wires:
  [inertia] -> Matrix Multiply14/1
  Matrix Multiply2/1 -> Radians to Degrees/1, Cross Product/1, Derivative1/1, Matrix Multiply15/2
  [hwheelsbody] -> Sum5/2
  Sum5/1 -> Cross Product/2
  Matrix Multiply14/1 -> Sum4/1
  Cross Product/1 -> Sum4/2
  Matrix Multiply15/1 -> Sum5/1
  Derivative1/1 -> Matrix Multiply14/2
  w_ref/1(ref) -> Matrix Multiply2/2
  [inertia] -> Matrix Multiply15/1
  DCM_icrf2b/1 -> Matrix Multiply2/1
  Vicrf/1 -> w_ref/2(Vicrf)
  Sum4/1 -> target_torque/1  "target_torque"
  Xicrf/1 -> w_ref/1(Xicrf)
  inertia/1 -> [inertia]
  hwheelsbody/1 -> [hwheelsbody]
  Radians to Degrees/1 -> ?

== system satellite_dynamics/Moving Averaage ==
  omega_in : Inport
  Demux4 : Demux  Outputs=3
  Moving Average : dspstat3/Moving Average  Method=Sliding window  ForgettingFactorPort=off  SpecifyWindowLength=on  WindowLength=single(Kalman.Ts/gyro.Ts)  OverlapLength=single(Kalman.Ts/gyro.Ts) - single(1)  AllowArbitraryInputLength=off  ForgettingFactor=0.9  SimulateUsing=Interpreted execution
  Moving Average1 : dspstat3/Moving Average  Method=Sliding window  ForgettingFactorPort=off  SpecifyWindowLength=on  WindowLength=single(Kalman.Ts/gyro.Ts)  OverlapLength=single(Kalman.Ts/gyro.Ts) - single(1)  AllowArbitraryInputLength=off  ForgettingFactor=0.9  SimulateUsing=Interpreted execution
  Moving Average2 : dspstat3/Moving Average  Method=Sliding window  ForgettingFactorPort=off  SpecifyWindowLength=on  WindowLength=single(Kalman.Ts/gyro.Ts)  OverlapLength=single(Kalman.Ts/gyro.Ts) - single(1)  AllowArbitraryInputLength=off  ForgettingFactor=0.9  SimulateUsing=Interpreted execution
  Mux2 : Mux  Inputs=3
  omega_movav : Outport
  wires:
  Mux2/1 -> omega_movav/1
  Moving Average2/1 -> Mux2/3
  omega_in/1 -> Demux4/1
  Demux4/3 -> Moving Average2/1
  Moving Average1/1 -> Mux2/2
  Demux4/1 -> Moving Average/1
  Demux4/2 -> Moving Average1/1
  Moving Average/1 -> Mux2/1

== system satellite_dynamics/Subsystem ==
  In1 : Inport
  In2 : Inport  Port=2
  Enable : EnablePort
  Bias : Bias  Bias=-1000 + 1e-6  SaturateOnIntegerOverflow=off
  Discrete-Time Integrator : DiscreteIntegrator  SampleTime=-1  ICPrevOutput=DiscIntNeverNeededParam  ICPrevScaledInput=DiscIntNeverNeededParam
  Divide : Product  Inputs=*/
  Out1 : Outport
  wires:
  In1/1 -> Discrete-Time Integrator/1
  Discrete-Time Integrator/1 -> Divide/1
  Divide/1 -> Out1/1
  In2/1 -> Bias/1
  Bias/1 -> Divide/2

== system satellite_dynamics/Subsystem1 ==
  q : Inport
  Compare To Constant : simulink/Logic and Bit Operations/Compare To Constant  relop=<  const=0  OutDataTypeStr=boolean
  Gain : Gain  Gain=-1
  Selector : Selector  InputPortWidth=4  IndexOptions=Index vector (dialog)  Indices=[1]  OutputSizes=1
  Switch : Switch  Criteria=u2 > Threshold  SaturateOnIntegerOverflow=off  InputSameDT=off
  q_out : Outport
  wires:
  q/1 -> Gain/1, Selector/1, Switch/3
  Switch/1 -> q_out/1
  Selector/1 -> Compare To Constant/1
  Compare To Constant/1 -> Switch/2
  Gain/1 -> Switch/1

== system satellite_dynamics/Subsystem2 ==
  q : Inport
  r : Inport  Port=2
  Quaternion Multiplication1 : aerolibutil/Quaternion Multiplication
  q*r : Outport
  wires:
  r/1 -> Quaternion Multiplication1/2
  q/1 -> Quaternion Multiplication1/1
  Quaternion Multiplication1/1 -> q*r/1

== system satellite_dynamics/Subsystem3 ==
  q_icrf2b_kalman : Inport
  r : Inport  Port=2
  Quaternion Inverse : aerolibutil/Quaternion Inverse
  Quaternion Multiplication : aerolibutil/Quaternion Multiplication
  q*r : Outport
  wires:
  Quaternion Inverse/1 -> Quaternion Multiplication/1
  q_icrf2b_kalman/1 -> Quaternion Inverse/1
  r/1 -> Quaternion Multiplication/2
  Quaternion Multiplication/1 -> q*r/1

== system satellite_dynamics/Subsystem4 ==
  In1 : Inport
  In2 : Inport  Port=2
  Enable : EnablePort
  Bias : Bias  Bias=-1000 + 1e-6  SaturateOnIntegerOverflow=off
  Discrete-Time Integrator : DiscreteIntegrator  SampleTime=-1  ICPrevOutput=DiscIntNeverNeededParam  ICPrevScaledInput=DiscIntNeverNeededParam
  Divide : Product  Inputs=*/
  Out1 : Outport
  wires:
  In1/1 -> Discrete-Time Integrator/1
  Discrete-Time Integrator/1 -> Divide/1
  Divide/1 -> Out1/1
  In2/1 -> Bias/1
  Bias/1 -> Divide/2

== system satellite_dynamics/Subsystem6 ==
  q_icrf2b_kalman : Inport
  r : Inport  Port=2
  Quaternion Inverse : aerolibutil/Quaternion Inverse
  Quaternion Multiplication : aerolibutil/Quaternion Multiplication
  Subsystem1 : Subsystem
  q*r : Outport
  wires:
  Quaternion Inverse/1 -> Quaternion Multiplication/1
  q_icrf2b_kalman/1 -> Quaternion Inverse/1
  r/1 -> Quaternion Multiplication/2
  Quaternion Multiplication/1 -> Subsystem1/1(q)
  Subsystem1/1(q_out) -> q*r/1

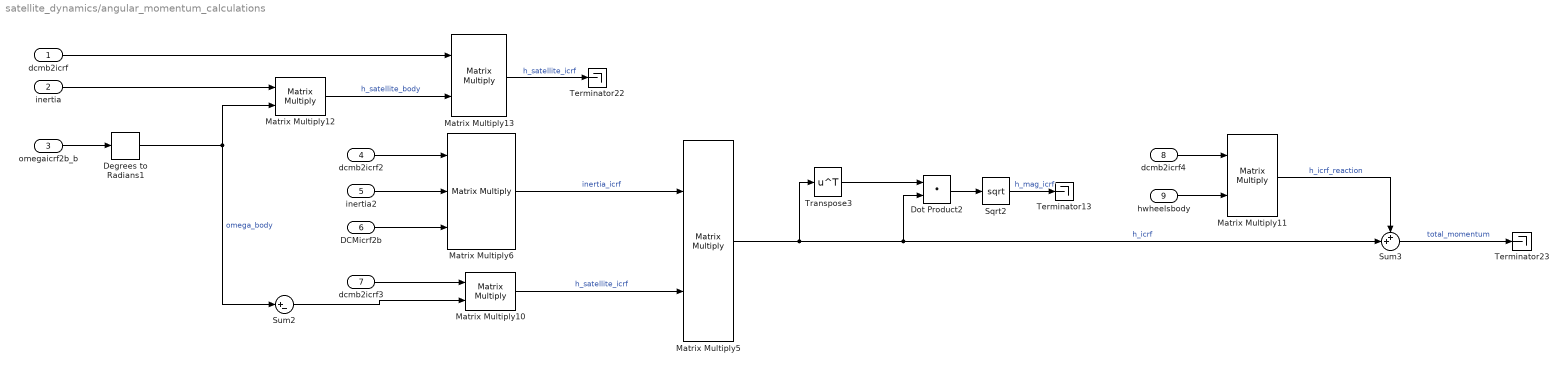
== system satellite_dynamics/angular_momentum_calculations ==
  dcmb2icrf : Inport
  inertia : Inport  Port=2
  omegaicrf2b_b : Inport  Port=3
  dcmb2icrf2 : Inport  Port=4
  inertia2 : Inport  Port=5
  DCMicrf2b : Inport  Port=6
  dcmb2icrf3 : Inport  Port=7
  dcmb2icrf4 : Inport  Port=8
  hwheelsbody : Inport  Port=9
  Degrees to Radians1 : simulink_extras/Transformations/Degrees to Radians
  Dot Product2 : DotProduct  OutDataTypeStr=Inherit: Inherit via internal rule
  Matrix Multiply{5,10..13} (5 alike) : Product  Multiplication=Matrix(*)
  Matrix Multiply6 : Product  Inputs=3  Multiplication=Matrix(*)
  Sqrt2 : Sqrt
  Sum2 : Sum  Inputs=|+-
  Sum3 : Sum  Inputs=++|
  Terminator13 : Terminator
  Terminator22 : Terminator
  Terminator23 : Terminator
  Transpose3 : Math  Operator=transpose
  wires:
  Degrees to Radians1/1 -> Matrix Multiply12/2, Sum2/1  "omega_body"
  Sqrt2/1 -> Terminator13/1  "h_mag_icrf"
  Matrix Multiply10/1 -> Matrix Multiply5/2  "h_satellite_icrf"
  Matrix Multiply12/1 -> Matrix Multiply13/2  "h_satellite_body"
  Sum2/1 -> Matrix Multiply10/2
  Dot Product2/1 -> Sqrt2/1
  Matrix Multiply11/1 -> Sum3/1  "h_icrf_reaction"
  Matrix Multiply6/1 -> Matrix Multiply5/1  "inertia_icrf"
  DCMicrf2b/1 -> Matrix Multiply6/3
  Transpose3/1 -> Dot Product2/1
  Matrix Multiply5/1 -> Transpose3/1, Sum3/2, Dot Product2/2  "h_icrf"
  Matrix Multiply13/1 -> Terminator22/1  "h_satellite_icrf"
  Sum3/1 -> Terminator23/1  "total_momentum"
  dcmb2icrf3/1 -> Matrix Multiply10/1
  inertia/1 -> Matrix Multiply12/1
  dcmb2icrf2/1 -> Matrix Multiply6/1
  dcmb2icrf4/1 -> Matrix Multiply11/1
  dcmb2icrf/1 -> Matrix Multiply13/1
  inertia2/1 -> Matrix Multiply6/2
  hwheelsbody/1 -> Matrix Multiply11/2
  omegaicrf2b_b/1 -> Degrees to Radians1/1

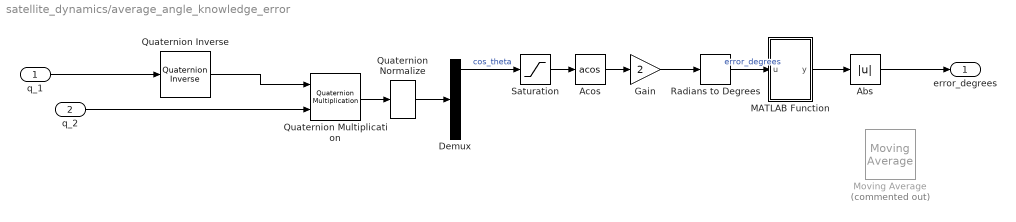
== system satellite_dynamics/average_angle_knowledge_error ==
  q_1 : Inport
  q_2 : Inport  Port=2
  Abs : Abs  SaturateOnIntegerOverflow=off
  Acos : Trigonometry  Operator=acos
  Demux : Demux
  Gain : Gain  Gain=2
  MATLAB Function : MATLAB Function  TreatAsAtomicUnit=on
  Moving Average : dspstat3/Moving Average  Commented=on  Method=Sliding window  ForgettingFactorPort=off  SpecifyWindowLength=on  WindowLength=samples  OverlapLength=samples - 1  AllowArbitraryInputLength=off  ForgettingFactor=0.9  SimulateUsing=Interpreted execution
  Quaternion Inverse : aerolibutil/Quaternion Inverse
  Quaternion Multiplication : aerolibutil/Quaternion Multiplication
  Quaternion Normalize : sharedutil/Quaternion Normalize  aMode=aMode
  Radians to Degrees : simulink_extras/Transformations/Radians to Degrees
  Saturation : Saturate  UpperLimit=1  LowerLimit=-1
  error_degrees : Outport
  wires:
  Gain/1 -> Radians to Degrees/1
  MATLAB Function/1(y) -> Abs/1
  Acos/1 -> Gain/1
  Saturation/1 -> Acos/1
  Quaternion Normalize/1 -> Demux/1
  Abs/1 -> error_degrees/1
  Radians to Degrees/1 -> MATLAB Function/1(u)  "error_degrees"
  Demux/1 -> Saturation/1  "cos_theta"
  Quaternion Multiplication/1 -> Quaternion Normalize/1
  Quaternion Inverse/1 -> Quaternion Multiplication/1
  q_2/1 -> Quaternion Multiplication/2
  q_1/1 -> Quaternion Inverse/1

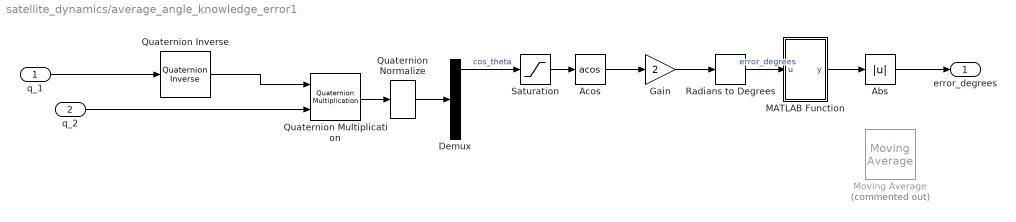
== system satellite_dynamics/average_angle_knowledge_error1 ==
  q_1 : Inport
  q_2 : Inport  Port=2
  Abs : Abs  SaturateOnIntegerOverflow=off
  Acos : Trigonometry  Operator=acos
  Demux : Demux
  Gain : Gain  Gain=2
  MATLAB Function : MATLAB Function  TreatAsAtomicUnit=on
  Moving Average : dspstat3/Moving Average  Commented=on  Method=Sliding window  ForgettingFactorPort=off  SpecifyWindowLength=on  WindowLength=samples  OverlapLength=samples - 1  AllowArbitraryInputLength=off  ForgettingFactor=0.9  SimulateUsing=Interpreted execution
  Quaternion Inverse : aerolibutil/Quaternion Inverse
  Quaternion Multiplication : aerolibutil/Quaternion Multiplication
  Quaternion Normalize : sharedutil/Quaternion Normalize  aMode=aMode
  Radians to Degrees : simulink_extras/Transformations/Radians to Degrees
  Saturation : Saturate  UpperLimit=1  LowerLimit=-1
  error_degrees : Outport
  wires:
  MATLAB Function/1(y) -> Abs/1
  Acos/1 -> Gain/1
  Saturation/1 -> Acos/1
  Quaternion Normalize/1 -> Demux/1
  Abs/1 -> error_degrees/1
  Radians to Degrees/1 -> MATLAB Function/1(u)  "error_degrees"
  Demux/1 -> Saturation/1  "cos_theta"
  Quaternion Multiplication/1 -> Quaternion Normalize/1
  Quaternion Inverse/1 -> Quaternion Multiplication/1
  q_2/1 -> Quaternion Multiplication/2
  q_1/1 -> Quaternion Inverse/1
  Gain/1 -> Radians to Degrees/1

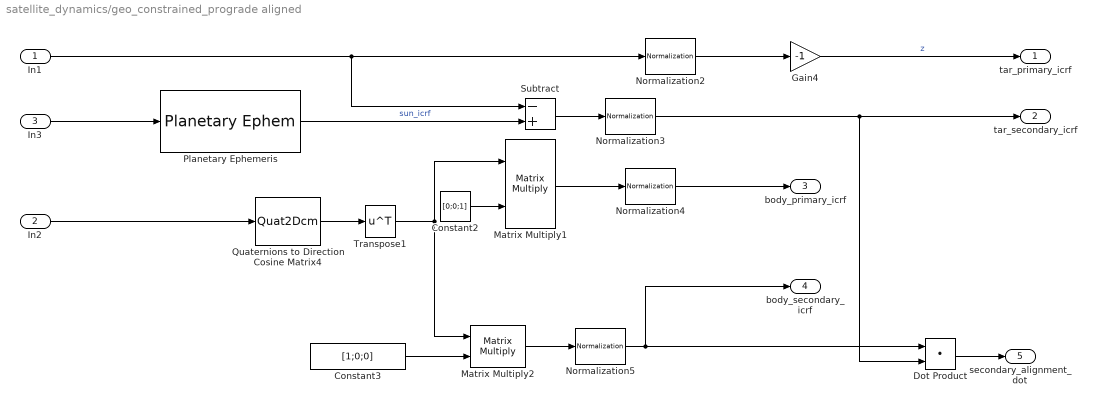
== system satellite_dynamics/geo_constrained_prograde aligned ==
  In1 : Inport
  In2 : Inport  Port=2
  In3 : Inport  Port=3
  Constant2 : Constant  Value=[0;0;1]
  Constant3 : Constant  Value=[1;0;0]
  Dot Product : DotProduct  OutDataTypeStr=Inherit: Inherit via internal rule
  Gain4 : Gain  Gain=-1
  Matrix Multiply1 : Product  Multiplication=Matrix(*)
  Matrix Multiply2 : Product  Multiplication=Matrix(*)
  Normalization{2..5} (4 alike) : dspmathops/Normalization  NormType=2-norm  Bias=1e-10  NormOver=Each column  Dimension=1  roundingMode=Floor  overflowMode=off  accumDataTypeStr=Inherit: Same as product output  accumLastDataTypeStr=Inherit: Same as product output  outputDataTypeStr=Inherit: Same as product output  outputMin=[]  outputMax=[]  outputLastDataTypeStr=Inherit: Same as product output
  Planetary Ephemeris : PlanetaryEphem  units=m,m/s  target=Sun  outputVelocity=off
  Quaternions to Direction Cosine Matrix4 : Quat2Dcm
  Subtract : Sum  Inputs=-+
  Transpose1 : Math  Operator=transpose
  tar_primary_icrf : Outport
  tar_secondary_icrf : Outport  Port=2
  body_primary_icrf : Outport  Port=3
  body_secondary_icrf : Outport  Port=4
  secondary_alignment_dot : Outport  Port=5
  wires:
  Subtract/1 -> Normalization3/1
  Matrix Multiply2/1 -> Normalization5/1
  Transpose1/1 -> Matrix Multiply2/1, Matrix Multiply1/1
  Normalization5/1 -> body_secondary_icrf/1, Dot Product/1
  In1/1 -> Subtract/1, Normalization2/1
  Normalization3/1 -> Dot Product/2, tar_secondary_icrf/1
  Quaternions to Direction Cosine Matrix4/1 -> Transpose1/1
  Planetary Ephemeris/1 -> Subtract/2  "sun_icrf"
  Dot Product/1 -> secondary_alignment_dot/1
  Constant3/1 -> Matrix Multiply2/2
  Matrix Multiply1/1 -> Normalization4/1
  Constant2/1 -> Matrix Multiply1/2
  Normalization2/1 -> Gain4/1
  Gain4/1 -> tar_primary_icrf/1  "z"
  Normalization4/1 -> body_primary_icrf/1
  In3/1 -> Planetary Ephemeris/1
  In2/1 -> Quaternions to Direction Cosine Matrix4/1

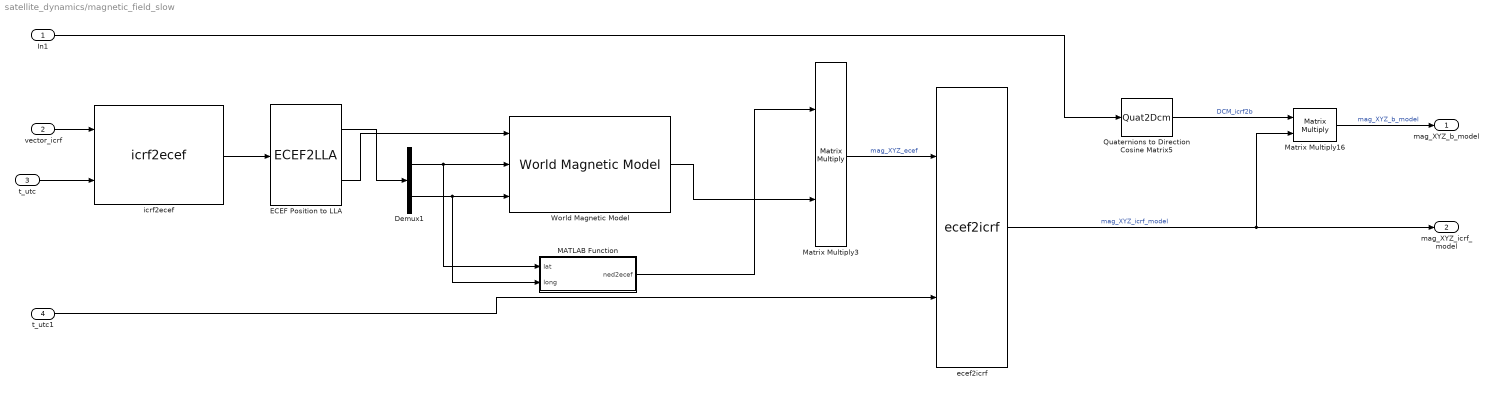
== system satellite_dynamics/magnetic_field_slow ==
  In1 : Inport
  vector_icrf : Inport  Port=2
  t_utc : Inport  Port=3
  t_utc1 : Inport  Port=4
  Demux1 : Demux  Outputs=2
  ECEF Position to LLA : ECEF2LLA
  MATLAB Function : MATLAB Function  TreatAsAtomicUnit=on
  Matrix Multiply16 : Product  Multiplication=Matrix(*)
  Matrix Multiply3 : Product  Multiplication=Matrix(*)
  Quaternions to Direction Cosine Matrix5 : Quat2Dcm
  World Magnetic Model : aerolibgravity2/World Magnetic Model  model=WMM2015 V2 (2015-2020)  customFile='WMM2025.COF'  units=Metric (MKS)  time_in=off  month=January  day=1  year=2020  action=Error  h_out=off  dec_out=off  inc_out=off  ti_out=off
  ecef2icrf : utilities/ecef2icrf  SystemSampleTime=-1  VariantActivationTime=update diagram  EmptyChoice=off  PassThrough=off  PassThroughVariantControl=(default)  EmptyChoiceVariantControl=(default)  AllowFlexibleInterface=on  Latency=0  AutoFrameSizeCalculation=off
  icrf2ecef : utilities/icrf2ecef  SystemSampleTime=-1  VariantActivationTime=update diagram  EmptyChoice=off  PassThrough=off  PassThroughVariantControl=(default)  EmptyChoiceVariantControl=(default)  AllowFlexibleInterface=on  Latency=0  AutoFrameSizeCalculation=off
  mag_XYZ_b_model : Outport
  mag_XYZ_icrf_model : Outport  Port=2
  wires:
  ecef2icrf/1 -> mag_XYZ_icrf_model/1, Matrix Multiply16/2  "mag_XYZ_icrf_model"
  World Magnetic Model/1 -> Matrix Multiply3/2
  Demux1/1 -> MATLAB Function/1(lat), World Magnetic Model/2
  icrf2ecef/1 -> ECEF Position to LLA/1
  MATLAB Function/1(ned2ecef) -> Matrix Multiply3/1
  Demux1/2 -> MATLAB Function/2(long), World Magnetic Model/3
  Quaternions to Direction Cosine Matrix5/1 -> Matrix Multiply16/1  "DCM_icrf2b"
  ECEF Position to LLA/2 -> World Magnetic Model/1
  Matrix Multiply3/1 -> ecef2icrf/1  "mag_XYZ_ecef"
  ECEF Position to LLA/1 -> Demux1/1
  In1/1 -> Quaternions to Direction Cosine Matrix5/1
  vector_icrf/1 -> icrf2ecef/1
  t_utc/1 -> icrf2ecef/2
  Matrix Multiply16/1 -> mag_XYZ_b_model/1  "mag_XYZ_b_model"
  t_utc1/1 -> ecef2icrf/2

== system satellite_dynamics/magtor_controller ==
  mag_XYZ_body : Inport
  h_wheels_body : Inport  Port=2
  Bias : Bias  Bias=-h_default  SaturateOnIntegerOverflow=off
  Cross Product : matrix_library/Cross Product
  Divide : Product  Inputs=*/
  Gain : Gain  Gain=mag_torque.k
  Gain1 : Gain  Gain=1e-9
  Gain2 : Gain  Gain=1/mag_torque.gain
  Normalization : dspmathops/Normalization  NormType=2-norm  Bias=1e-10  NormOver=Each column  Dimension=1  roundingMode=Floor  overflowMode=off  accumDataTypeStr=Inherit: Same as product output  accumLastDataTypeStr=Inherit: Same as product output  outputDataTypeStr=Inherit: Same as product output  outputMin=[]  outputMax=[]  outputLastDataTypeStr=Inherit: Same as product output
  vector_magnitude : utilities/vector_magnitude
  currents : Outport
  wires:
  mag_XYZ_body/1 -> Gain1/1, Normalization/1
  Normalization/1 -> Cross Product/2
  h_wheels_body/1 -> Bias/1
  Cross Product/1 -> Gain/1
  Gain/1 -> Divide/1
  vector_magnitude/1 -> Divide/2
  Gain1/1 -> vector_magnitude/1
  Divide/1 -> Gain2/1  "dipole_command"
  Gain2/1 -> currents/1
  Bias/1 -> Cross Product/1

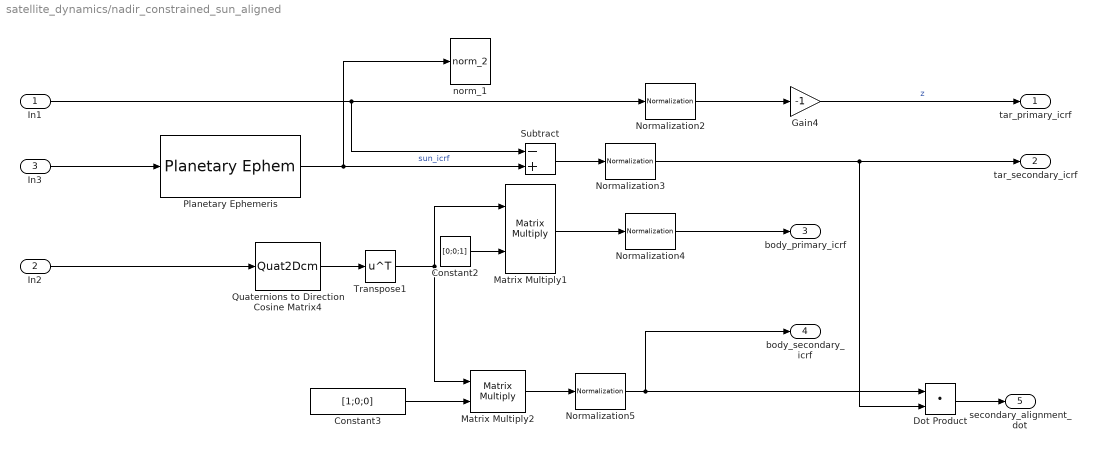
== system satellite_dynamics/nadir_constrained_sun_aligned ==
  In1 : Inport
  In2 : Inport  Port=2
  In3 : Inport  Port=3
  Constant2 : Constant  Value=[0;0;1]
  Constant3 : Constant  Value=[1;0;0]
  Dot Product : DotProduct  OutDataTypeStr=Inherit: Inherit via internal rule
  Gain4 : Gain  Gain=-1
  Matrix Multiply1 : Product  Multiplication=Matrix(*)
  Matrix Multiply2 : Product  Multiplication=Matrix(*)
  Normalization{2..5} (4 alike) : dspmathops/Normalization  NormType=2-norm  Bias=1e-10  NormOver=Each column  Dimension=1  roundingMode=Floor  overflowMode=off  accumDataTypeStr=Inherit: Same as product output  accumLastDataTypeStr=Inherit: Same as product output  outputDataTypeStr=Inherit: Same as product output  outputMin=[]  outputMax=[]  outputLastDataTypeStr=Inherit: Same as product output
  Planetary Ephemeris : PlanetaryEphem  units=m,m/s  target=Sun  outputVelocity=off
  Quaternions to Direction Cosine Matrix4 : Quat2Dcm
  Subtract : Sum  Inputs=-+
  Transpose1 : Math  Operator=transpose
  norm_1 : utilities/norm_2  SystemSampleTime=-1  SSRTWFcnClass=[]  VariantActivationTime=update diagram  EmptyChoice=off  PassThrough=off  PassThroughVariantControl=(default)  EmptyChoiceVariantControl=(default)  AllowFlexibleInterface=on  Latency=0  AutoFrameSizeCalculation=off
  tar_primary_icrf : Outport
  tar_secondary_icrf : Outport  Port=2
  body_primary_icrf : Outport  Port=3
  body_secondary_icrf : Outport  Port=4
  secondary_alignment_dot : Outport  Port=5
  wires:
  Subtract/1 -> Normalization3/1
  Matrix Multiply2/1 -> Normalization5/1
  Transpose1/1 -> Matrix Multiply2/1, Matrix Multiply1/1
  Normalization5/1 -> body_secondary_icrf/1, Dot Product/1
  In1/1 -> Subtract/1, Normalization2/1
  Normalization3/1 -> Dot Product/2, tar_secondary_icrf/1
  Quaternions to Direction Cosine Matrix4/1 -> Transpose1/1
  Planetary Ephemeris/1 -> norm_1/1, Subtract/2  "sun_icrf"
  Dot Product/1 -> secondary_alignment_dot/1
  Constant3/1 -> Matrix Multiply2/2
  Matrix Multiply1/1 -> Normalization4/1
  Constant2/1 -> Matrix Multiply1/2
  Normalization2/1 -> Gain4/1
  Gain4/1 -> tar_primary_icrf/1  "z"
  Normalization4/1 -> body_primary_icrf/1
  In3/1 -> Planetary Ephemeris/1
  In2/1 -> Quaternions to Direction Cosine Matrix4/1

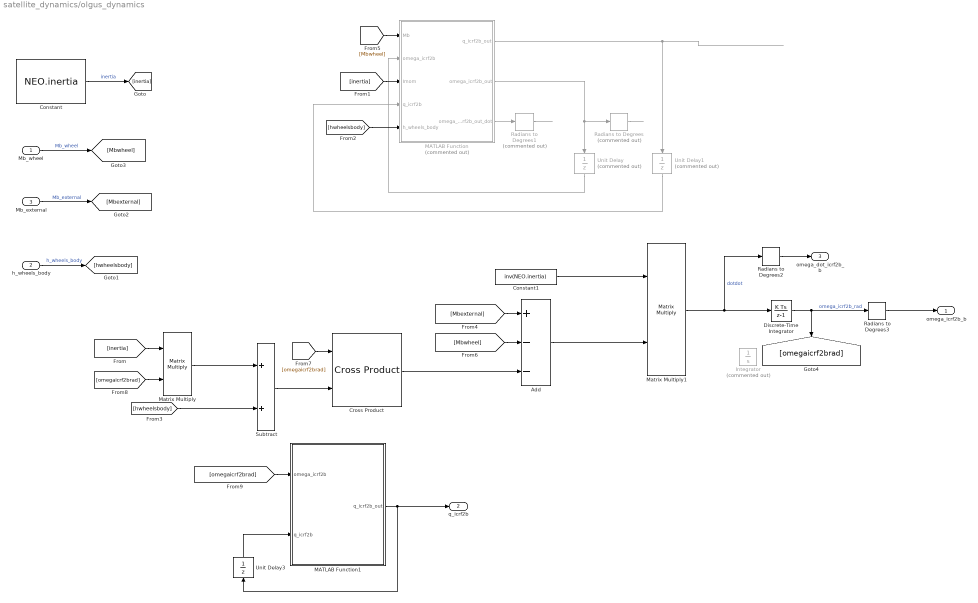
== system satellite_dynamics/olgus_dynamics ==
  Mb_wheel : Inport
  h_wheels_body : Inport  Port=2
  Mb_external : Inport  Port=3
  Add : Sum  Inputs=+--
  Constant : Constant  Value=NEO.inertia
  Constant1 : Constant  Value=inv(NEO.inertia)
  Cross Product : matrix_library/Cross Product
  Discrete-Time Integrator : DiscreteIntegrator  InitialCondition=deg2rad(omega_icrf2b_initial)  SampleTime=-1  ICPrevOutput=DiscIntNeverNeededParam  ICPrevScaledInput=DiscIntNeverNeededParam
  Integrator : Integrator  Commented=on  InitialCondition=deg2rad(omega_icrf2b_initial)
  MATLAB Function : MATLAB Function  Commented=on  TreatAsAtomicUnit=on
  MATLAB Function1 : MATLAB Function  TreatAsAtomicUnit=on
  Matrix Multiply : Product  Multiplication=Matrix(*)
  Matrix Multiply1 : Product  Multiplication=Matrix(*)
  Radians to Degrees : simulink_extras/Transformations/Radians to Degrees  Commented=on
  Radians to Degrees1 : simulink_extras/Transformations/Radians to Degrees  Commented=on
  Radians to Degrees2 : simulink_extras/Transformations/Radians to Degrees
  Radians to Degrees3 : simulink_extras/Transformations/Radians to Degrees
  Subtract : Sum
  Unit Delay : UnitDelay  Commented=on  InitialCondition=deg2rad(omega_icrf2b_initial)  SampleTime=-1  HasFrameUpgradeWarning=on
  Unit Delay1 : UnitDelay  Commented=on  InitialCondition=q_icrf2b_initial  SampleTime=-1  HasFrameUpgradeWarning=on
  Unit Delay3 : UnitDelay  InitialCondition=q_icrf2b_initial  SampleTime=-1  HasFrameUpgradeWarning=on
  omega_icrf2b_b : Outport
  q_icrf2b : Outport  Port=2
  omega_dot_icrf2b_b : Outport  Port=3
  wires:
  MATLAB Function/1(q_icrf2b_out) -> Unit Delay1/1
  MATLAB Function/2(omega_icrf2b_out) -> Radians to Degrees/1, Unit Delay/1
  Unit Delay/1 -> MATLAB Function/2(omega_icrf2b)
  Unit Delay1/1 -> MATLAB Function/4(q_icrf2b)
  Radians to Degrees/1 -> ?
  MATLAB Function/3(omega_icrf2b_out_dot) -> Radians to Degrees1/1
  Radians to Degrees1/1 -> ?
  Add/1 -> Matrix Multiply1/2
  Matrix Multiply/1 -> Subtract/1
  Subtract/1 -> Cross Product/2
  Cross Product/1 -> Add/3
  Constant1/1 -> Matrix Multiply1/1
  Matrix Multiply1/1 -> Discrete-Time Integrator/1, Radians to Degrees2/1  "dotdot"
  Discrete-Time Integrator/1 -> Radians to Degrees3/1, [omegaicrf2brad]  "omega_icrf2b_rad"
  Radians to Degrees2/1 -> omega_dot_icrf2b_b/1
  Radians to Degrees3/1 -> omega_icrf2b_b/1
  Unit Delay3/1 -> MATLAB Function1/2(q_icrf2b)
  MATLAB Function1/1(q_icrf2b_out) -> Unit Delay3/1, q_icrf2b/1
  Constant/1 -> [inertia]  "inertia"
  [inertia] -> Matrix Multiply/1
  [inertia] -> MATLAB Function/3(Imom)
  h_wheels_body/1 -> [hwheelsbody]  "h_wheels_body"
  [hwheelsbody] -> MATLAB Function/5(h_wheels_body)
  [hwheelsbody] -> Subtract/2
  Mb_external/1 -> [Mbexternal]  "Mb_external"
  [Mbexternal] -> Add/1
  Mb_wheel/1 -> [Mbwheel]  "Mb_wheel"
  [Mbwheel] -> MATLAB Function/1(Mb)
  [Mbwheel] -> Add/2
  [omegaicrf2brad] -> Cross Product/1
  [omegaicrf2brad] -> Matrix Multiply/2
  [omegaicrf2brad] -> MATLAB Function1/1(omega_icrf2b)

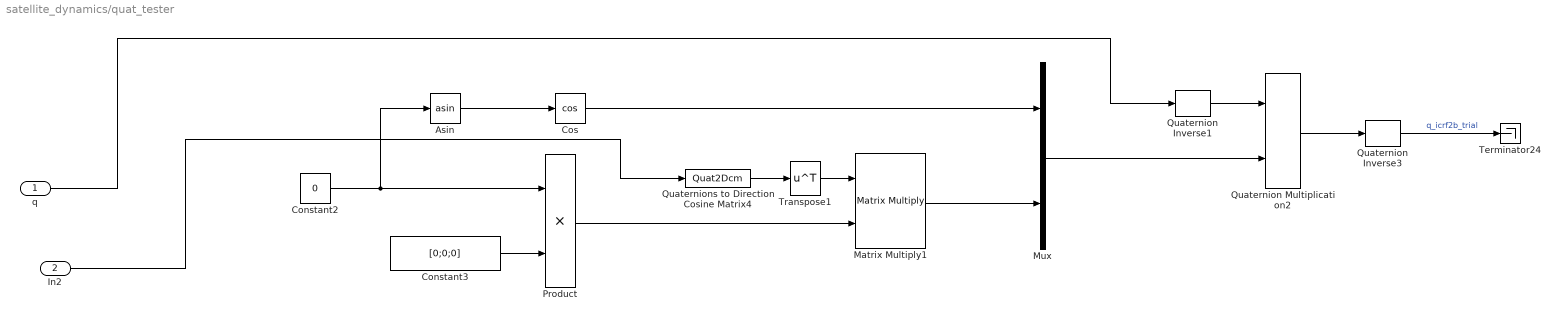
== system satellite_dynamics/quat_tester ==
  q : Inport
  In2 : Inport  Port=2
  Asin : Trigonometry  Operator=asin
  Constant2 : Constant  Value=0
  Constant3 : Constant  Value=[0;0;0]
  Cos : Trigonometry  Operator=cos
  Matrix Multiply1 : Product  Multiplication=Matrix(*)
  Mux : Mux  Inputs=2
  Product : Product
  Quaternion Inverse1 : aerolibutil/Quaternion Inverse
  Quaternion Inverse3 : aerolibutil/Quaternion Inverse
  Quaternion Multiplication2 : aerolibutil/Quaternion Multiplication
  Quaternions to Direction Cosine Matrix4 : Quat2Dcm
  Terminator24 : Terminator
  Transpose1 : Math  Operator=transpose
  wires:
  Mux/1 -> Quaternion Multiplication2/2
  Quaternion Multiplication2/1 -> Quaternion Inverse3/1
  Matrix Multiply1/1 -> Mux/2
  Transpose1/1 -> Matrix Multiply1/1
  Asin/1 -> Cos/1
  Quaternion Inverse3/1 -> Terminator24/1  "q_icrf2b_trial"
  Constant2/1 -> Asin/1, Product/1
  Quaternions to Direction Cosine Matrix4/1 -> Transpose1/1
  Cos/1 -> Mux/1
  Constant3/1 -> Product/2
  Quaternion Inverse1/1 -> Quaternion Multiplication2/1
  Product/1 -> Matrix Multiply1/2
  q/1 -> Quaternion Inverse1/1
  In2/1 -> Quaternions to Direction Cosine Matrix4/1

== system satellite_dynamics/quat_tester_2 ==
  In1 : Inport
  X_icrf : Inport  Port=2
  Constant1 : Constant  Value=[0;0;1]
  Dot Product : DotProduct  OutDataTypeStr=Inherit: Inherit via internal rule
  Integrator2 : Integrator
  Matrix Multiply : Product  Multiplication=Matrix(*)
  Normalization : dspmathops/Normalization  NormType=2-norm  Bias=1e-10  NormOver=Each column  Dimension=1  roundingMode=Floor  overflowMode=off  accumDataTypeStr=Inherit: Same as product output  accumLastDataTypeStr=Inherit: Same as product output  outputDataTypeStr=Inherit: Same as product output  outputMin=[]  outputMax=[]  outputLastDataTypeStr=Inherit: Same as product output
  Normalization1 : dspmathops/Normalization  NormType=2-norm  Bias=1e-10  NormOver=Each column  Dimension=1  roundingMode=Floor  overflowMode=off  accumDataTypeStr=Inherit: Same as product output  accumLastDataTypeStr=Inherit: Same as product output  outputDataTypeStr=Inherit: Same as product output  outputMin=[]  outputMax=[]  outputLastDataTypeStr=Inherit: Same as product output
  Quaternions to Direction Cosine Matrix3 : Quat2Dcm
  Terminator13 : Terminator
  Terminator22 : Terminator
  Transpose : Math  Operator=transpose
  wires:
  Transpose/1 -> Matrix Multiply/1
  Matrix Multiply/1 -> Normalization/1
  Dot Product/1 -> Terminator13/1
  Normalization/1 -> Dot Product/1
  Normalization1/1 -> Integrator2/1, Dot Product/2
  Integrator2/1 -> Terminator22/1
  Constant1/1 -> Matrix Multiply/2
  Quaternions to Direction Cosine Matrix3/1 -> Transpose/1
  X_icrf/1 -> Normalization1/1
  In1/1 -> Quaternions to Direction Cosine Matrix3/1
